simulink model "VesselSimulator"  (R2016a)
settings: Solver=FixedStepAuto  StartTime=0.0  StopTime=inf  FixedStep=0.05  RelTol=1e-3
undefined symbols (not defined in the file or in its folder): C_nuParams, D, D_nuParams, invM, MAPP1, MAPP2, MAPP3, Th1, Th2, Th3, Tr, X, Y, Z
libraries: robotlib x5, realtime_pacer_lib x1
settings Model: Creator=einar  LastModifiedBy=einar
settings DataIOCC: LimitDataPoints=on
settings OptimizationCC: OptimizeModelRefInitCode=on  LifeSpan=Inf  MaxStackSize=64
settings DebuggingCC: AllowSymbolicDim=off
settings HardwareCC: ProdBitPerPointer=32  ProdLargestAtomicFloat=None  ProdIntDivRoundTo=Undefined  ProdEndianess=Unspecified  ProdWordSize=32  ProdHWDeviceType=Generic->Unspecified (assume 32-bit Generic)
settings ModelReferenceCC: PropagateSignalLabelsOutOfModel=off
settings RTWCC: SystemTargetFile=ert.tlc  HardwareBoard=Robot Operating System (ROS)  TemplateMakefile=ert_default_tmf  Toolchain=Catkin  TargetLang=C++
settings CodeAppCC: IgnoreCustomStorageClasses=off
settings ERTTargetCC: SupportContinuousTime=on  ConvertIfToSwitch=off  SuppressUnreachableDefaultCases=off

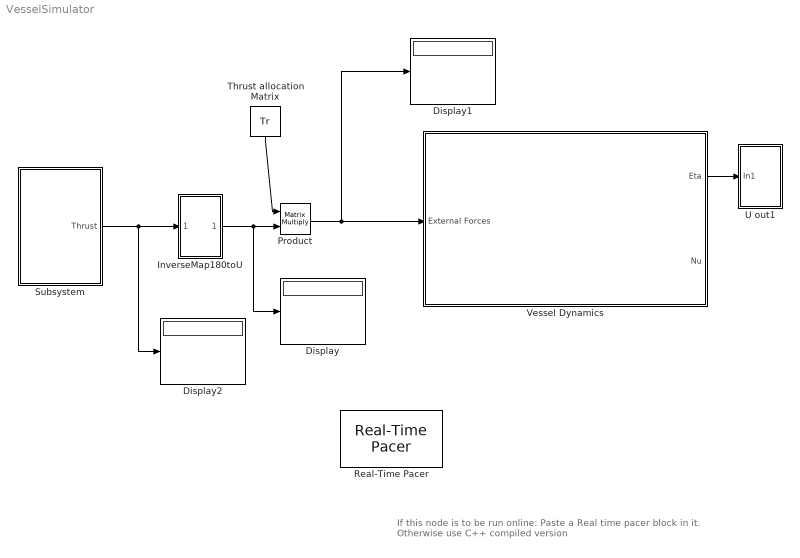
== system VesselSimulator ==
  note: If this node is to be run online: Paste a Real time pacer block in it.
      | Otherwise use C++ compiled version
  Display : Display
  Display1 : Display
  Display2 : Display
  InverseMap180toU : Subsystem
  Product : Product  Multiplication=Matrix(*)
  Real-Time Pacer : realtime_pacer_lib/Real-Time Pacer  simTimePerRealTime=1
  Subsystem : Subsystem
  Thrust allocation Matrix : Constant  Value=Tr
  U out1 : Subsystem
  Vessel Dynamics : Subsystem
  wires:
  Thrust allocation Matrix/1 -> Product/1
  Product/1 -> Display1/1, Vessel Dynamics/1(External Forces)
  Vessel Dynamics/1("Eta ") -> U out1/1(In1)
  Subsystem/1("Thrust ") -> Display2/1, InverseMap180toU/1(In1)
  InverseMap180toU/1(Out1) -> Display/1, Product/2

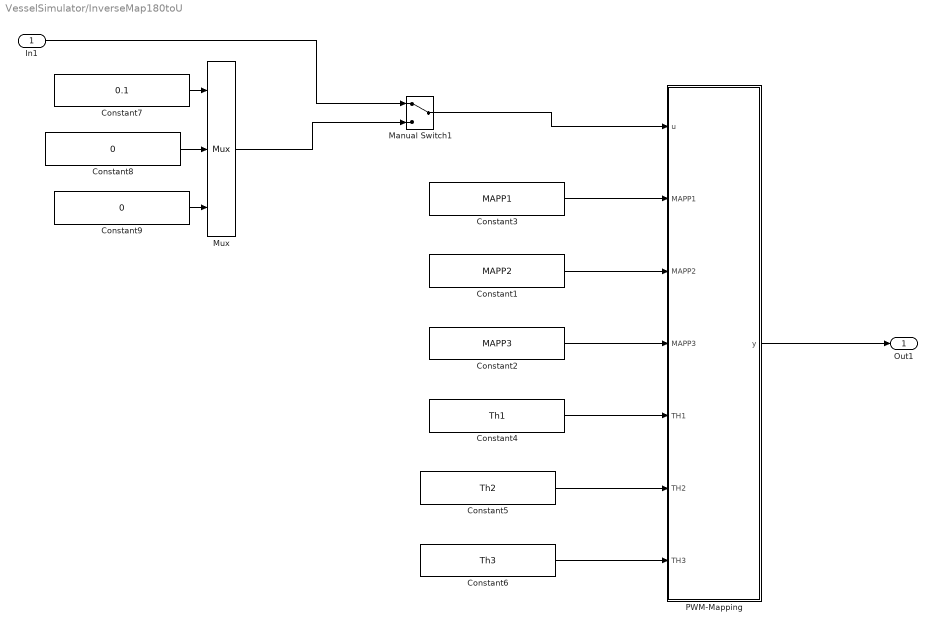
== system VesselSimulator/InverseMap180toU ==
  In1 : Inport
  Constant1 : Constant  Value=MAPP2
  Constant2 : Constant  Value=MAPP3
  Constant3 : Constant  Value=MAPP1
  Constant4 : Constant  Value=Th1
  Constant5 : Constant  Value=Th2
  Constant6 : Constant  Value=Th3
  Constant7 : Constant  Value=0.1
  Constant8 : Constant  Value=0
  Constant9 : Constant  Value=0
  Manual Switch1 : ManualSwitch
  Mux : Mux  Inputs=3
  PWM-Mapping : MATLAB Function  TreatAsAtomicUnit=on
  Out1 : Outport
  wires:
  Constant9/1 -> Mux/3
  Mux/1 -> Manual Switch1/2
  Constant8/1 -> Mux/2
  Constant7/1 -> Mux/1
  In1/1 -> Manual Switch1/1
  PWM-Mapping/1(y) -> Out1/1
  Constant2/1 -> PWM-Mapping/4(MAPP3)
  Constant1/1 -> PWM-Mapping/3(MAPP2)
  Constant3/1 -> PWM-Mapping/2(MAPP1)
  Constant5/1 -> PWM-Mapping/6(TH2)
  Constant6/1 -> PWM-Mapping/7(TH3)
  Constant4/1 -> PWM-Mapping/5(TH1)
  Manual Switch1/1 -> PWM-Mapping/1(u)

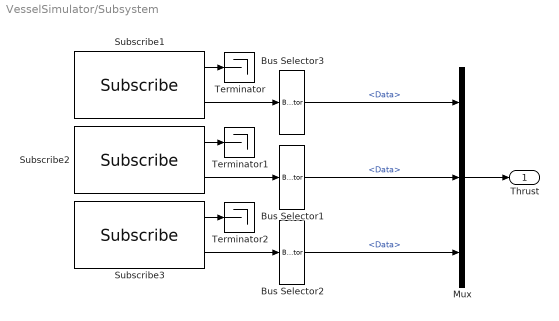
== system VesselSimulator/Subsystem ==
  Bus Selector1 : BusSelector  OutputSignals=Data
  Bus Selector2 : BusSelector  OutputSignals=Data
  Bus Selector3 : BusSelector  OutputSignals=Data
  Mux : Mux  Inputs=3
  Subscribe1 : robotlib/Subscribe  SourceLibraryInfo=This block requires Robotics System Toolbox  topicSource=Select from ROS network  topic=/Thrust1  messageType=std_msgs/UInt16  sampleTime=-1  messageQueueLength=1
  Subscribe2 : robotlib/Subscribe  SourceLibraryInfo=This block requires Robotics System Toolbox  topicSource=Select from ROS network  topic=/Thrust2  messageType=std_msgs/UInt16  sampleTime=-1  messageQueueLength=1
  Subscribe3 : robotlib/Subscribe  SourceLibraryInfo=This block requires Robotics System Toolbox  topicSource=Select from ROS network  topic=/Thrust3  messageType=std_msgs/UInt16  sampleTime=-1  messageQueueLength=1
  Terminator : Terminator
  Terminator1 : Terminator
  Terminator2 : Terminator
  "Thrust " : Outport
  wires:
  Mux/1 -> "Thrust "/1
  Subscribe1/1 -> Terminator/1
  Bus Selector3/1 -> Mux/1  "<Data>"
  Bus Selector1/1 -> Mux/2  "<Data>"
  Bus Selector2/1 -> Mux/3  "<Data>"
  Subscribe2/1 -> Terminator1/1
  Subscribe3/2 -> Bus Selector2/1
  Subscribe2/2 -> Bus Selector1/1
  Subscribe1/2 -> Bus Selector3/1
  Subscribe3/1 -> Terminator2/1

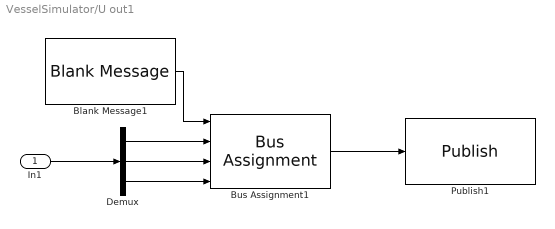
== system VesselSimulator/U out1 ==
  In1 : Inport
  Blank Message1 : robotlib/Blank Message  SourceLibraryInfo=This block requires Robotics System Toolbox  messageType=geometry_msgs/Vector3  SampleTime=inf
  Bus Assignment1 : BusAssignment  AssignedSignals=X,Y,Z
  Demux : Demux  Outputs=3
  Publish1 : robotlib/Publish  SourceLibraryInfo=This block requires Robotics System Toolbox  topicSource=Select from ROS network  topic=/Position  messageType=geometry_msgs/Vector3  messageQueueLength=1
  wires:
  Bus Assignment1/1 -> Publish1/1
  Blank Message1/1 -> Bus Assignment1/1
  In1/1 -> Demux/1
  Demux/1 -> Bus Assignment1/2
  Demux/3 -> Bus Assignment1/4
  Demux/2 -> Bus Assignment1/3

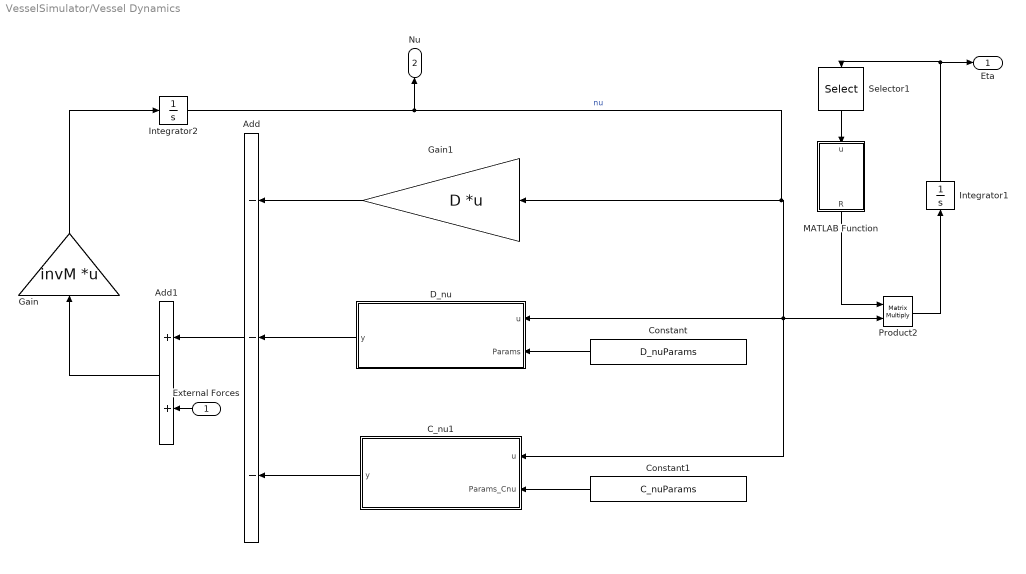
== system VesselSimulator/Vessel Dynamics ==
  External Forces : Inport
  Add : Sum  Inputs=---
  Add1 : Sum
  C_nu1 : MATLAB Function  TreatAsAtomicUnit=on
  Constant : Constant  Value=D_nuParams
  Constant1 : Constant  Value=C_nuParams
  D_nu : MATLAB Function  TreatAsAtomicUnit=on
  Gain : Gain  Gain=invM  Multiplication=Matrix(K*u) (u vector)
  Gain1 : Gain  Gain=D  Multiplication=Matrix(K*u) (u vector)
  Integrator1 : Integrator  InitialCondition=[0;0;0]
  Integrator2 : Integrator  InitialCondition=[0; 0; 0]
  MATLAB Function : MATLAB Function  TreatAsAtomicUnit=on
  Product2 : Product  Multiplication=Matrix(*)
  Selector1 : Selector  InputPortWidth=3  IndexOptions=Index vector (dialog)  Indices=[3]  OutputSizes=1
  "Eta " : Outport
  Nu : Outport  Port=2
  wires:
  External Forces/1 -> Add1/2
  Gain1/1 -> Add/1
  D_nu/1(y) -> Add/2
  Gain/1 -> Integrator2/1
  Constant/1 -> D_nu/2(Params)
  Product2/1 -> Integrator1/1
  Integrator1/1 -> Selector1/1, "Eta "/1
  Constant1/1 -> C_nu1/2(Params_Cnu)
  MATLAB Function/1(R) -> Product2/1
  Add/1 -> Add1/1
  C_nu1/1(y) -> Add/3
  Integrator2/1 -> Product2/2, C_nu1/1(u), D_nu/1(u), Gain1/1, Nu/1  "nu"
  Selector1/1 -> MATLAB Function/1(u)
  Add1/1 -> Gain/1

== matlab function VesselSimulator/InverseMap180toU/PWM-Mapping ==
  data: u input; y output; MAPP1 input; MAPP2 input; MAPP3 input; TH1 input; TH2 input; TH3 input
function y = fcn(u,MAPP1,MAPP2,MAPP3,TH1,TH2,TH3)
%load matrix mapperMat prior to running this node
y=[0 ;0;0];
for i=1:3
    if (u(i))==0
        u(i)=80;
    end
end
u(3)=-u(3);
TH3=-TH1;
MAPP3=MAPP1;

if u(1)>max(TH1)
    u(1)=max(TH1)
elseif u(1)<min(TH1)
u(1)=min(TH1);
end

if u(2)>max(TH2)
    u(2)=max(TH2);
elseif u(2)<min(TH2)
u(2)=min(TH2);
end

if u(3)>max(TH3)
    u(3)=max(TH3);
elseif u(3)<min(TH3)
u(3)=min(TH3);
end

y(1)=interp1(TH1,MAPP1,u(1));
y(2)=interp1(TH2,MAPP2,u(2));
y(3)=interp1(TH3,MAPP3,u(3));

if abs(u(1))<0.01
    y(1)=80;
end
if abs(u(2))<0.01
    y(2)=80;
end
if abs(u(3))<0.01
    y(3)=80;
end
for i=1:3
    if abs(y(i))<0.01
        y(i)=0;
    end
end

== matlab function VesselSimulator/Vessel Dynamics/D_nu ==
  data: u input; y output; Params input
function y = fcn(u,Params)
%#codegen
Dnu=[Params(1,1)*abs(u(1)) 0 0;0 Params(2,2)*abs(u(2)) 0;0 0 0];
y=Dnu*u;

== matlab function VesselSimulator/Vessel Dynamics/C_nu1 ==
  data: u input; y output; Params_Cnu input
function y = fcn(u,Params_Cnu)
%#codegen
C=[0 Params_Cnu(1,2)*u(3) 0;Params_Cnu(2,1)*u(3) 0 0;0 0 0];
y=C*u;

== matlab function VesselSimulator/Vessel Dynamics/MATLAB Function ==
  data: u input; R output
function R = fcn(u)
R=[cos(u) -sin(u) 0;sin(u) cos(u) 0 ;0 0 1];
%R=[RotPhi(1:2,:);[0 0 0;0 0 0;0 0 0];RotPhi(3,:)]
end
